simulink model "VoiceTransmissionBaseband"  (R2018a)
settings: Solver=VariableStepAuto  StartTime=0.0  StopTime=6  RelTol=1e-3
libraries: dspmathops x3, commanabbnd3 x2, dspvision x2, phasedtxrxlib x2, commchan3 x1, dspsnks4 x1, commrflib2 x1
settings Model: Creator=ASUS  LastModifiedBy=ASUS

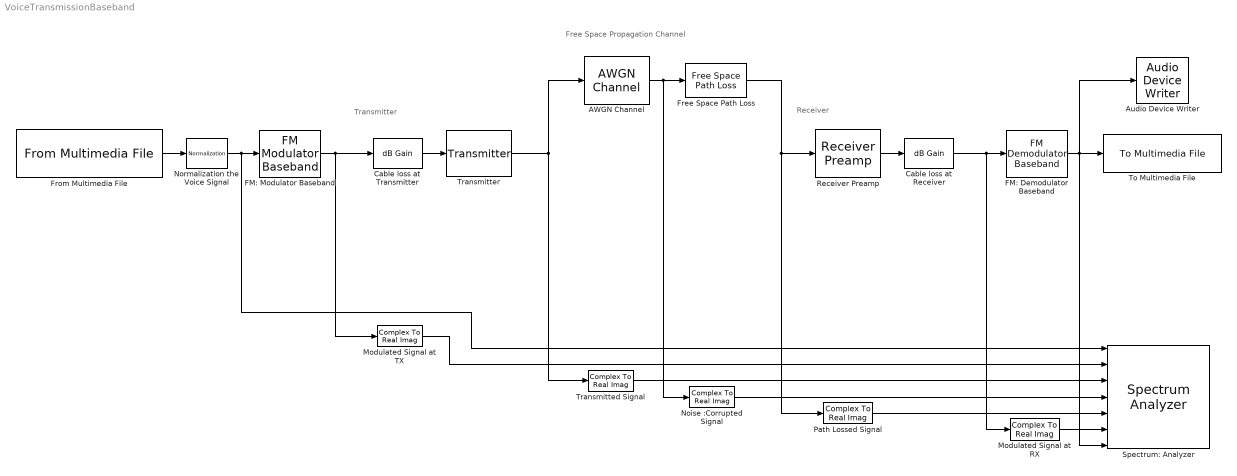
== system VoiceTransmissionBaseband ==
  note: Free Space Propagation Channel
  note: Receiver
  note: Transmitter
  AWGN Channel : commchan3/AWGN Channel  InputProcessing=Columns as channels (frame based)  seed=67  noiseMode="Signal to noise ratio  (Eb/No)"  EbNodB=-5  EsNodB=10  SNRdB=10  bitsPerSym=1  Ps=1  Tsym=1  variance=1
  Audio Device Writer : dspsnks4/Audio Device Writer  Driver=DirectSound  Device=Default  InheritSampleRate=on  SampleRate=44100  BitDepth=16-bit integer  BufferSize=4096  NumBuffers=10  DefaultOutputChannelMapping=on  OutputChannelMapping=1:2  OutputNumUnderrunSamples=off  DriverIdx=1  DeviceWarnFlag=''
  Cable loss at Receiver : dspmathops/dB Gain  dB=-4  intype=Amplitude
      settings: SourceProductName=DSP System Toolbox  SourceProductBaseCode=DS
  Cable loss at Transmitter : dspmathops/dB Gain  dB=-3  intype=Amplitude
      settings: SourceProductName=DSP System Toolbox  SourceProductBaseCode=DS
  "FM: Demodulator Baseband " : commanabbnd3/FM Demodulator Baseband   FrequencyDeviation=3999  SimulateUsing=Interpreted execution
      settings: SourceProductName=Communications System Toolbox  SourceProductBaseCode=CM
  FM: Modulator Baseband : commanabbnd3/FM Modulator Baseband  FrequencyDeviation=3999  SimulateUsing=Interpreted execution
      settings: SourceProductName=Communications System Toolbox  SourceProductBaseCode=CM
  Free Space Path Loss : commrflib2/Free Space Path Loss  mode=Decibels  dB=214.624  d=0.100  fc=1920
      settings: SourceProductName=Communications System Toolbox  SourceProductBaseCode=CM
  From Multimedia File : dspvision/From Multimedia File  inputFilename=C:\Users\ASUS\Desktop\GitRepos\RF-Propagation-Model\RFPL Modelling\code\voice.wav  loop=on  numPlays=inf  outputStreams=Audio only  videoDataType=single  audioDataType=double  inheritSampleTime=on  userDefinedSampleTime=1/30  noAudioOutput=off  isIntensityVideo=off  fourcc=RGB  colorVideoFormat=Separate color signals  outputEOF=off  dataOrg=Column-major  audioFrameSize=1024  computeAudioFrameSize=off  outSamplingMode=Sample based
      settings: SourceProductBaseCode=VP
  Modulated Signal at TX : ComplexToRealImag  Output=Real
  Modulated Signal at RX : ComplexToRealImag  Output=Real
  Noise :Corrupted Signal : ComplexToRealImag  Output=Real
  Normalization the Voice Signal : dspmathops/Normalization  NormType=2-norm  Bias=1e-10  NormOver=Each column  Dimension=1  roundingMode=Floor  overflowMode=off  accumDataTypeStr=Inherit: Same as product output  accumLastDataTypeStr=Inherit: Same as product output  outputDataTypeStr=Inherit: Same as product output  outputMin=[]  outputMax=[]  outputLastDataTypeStr=Inherit: Same as product output
      settings: SourceProductName=DSP System Toolbox
  Path Lossed Signal : ComplexToRealImag  Output=Real
  Receiver Preamp : phasedtxrxlib/Receiver Preamp  Gain=24.77  LossFactor=0  NoiseMethod=Noise temperature  NoiseFigure=0  ReferenceTemperature=290  SampleRateFromInputCheckbox=on  SampleRate=1e6  NoisePower=0  EnableInputPort=off  PhaseNoiseInputPort=off  SeedSource=Property  Seed=randi(65535,1)  SimulateUsing=Interpreted execution
      settings: SourceProductName=Phased Array System Toolbox  SourceProductBaseCode=AR
  Spectrum: Analyzer : SpectrumAnalyzer  NumInputPorts=7
  To Multimedia File : dspvision/To Multimedia File  outputFilename=C:\Users\ASUS\Desktop\GitRepos\RF-Propagation-Model\RFPL Modelling\code\output.wav  streamSelection=Audio only  videoCompressor=None (uncompressed)  audioCompressor=None (uncompressed)  imagePorts=Separate color signals  fileType=WAV  audioDatatype=16-bit integer  fourcc=RGB  videoQuality=75  mj2000CompFactor=10
      settings: SourceProductName=Computer Vision System Toolbox  SourceProductBaseCode=VP
  "Transmitted Signal " : ComplexToRealImag  Output=Real
  Transmitter : phasedtxrxlib/Transmitter  PeakPower=50000  Gain=30  LossFactor=0  InUseOutputPort=off  CoherentOnTransmit=on  PhaseNoiseOutputPort=off  SeedSource=Property  Seed=randi(65535,1)  SimulateUsing=Interpreted execution
      settings: SourceProductName=Phased Array System Toolbox  SourceProductBaseCode=AR
  wires:
  FM: Modulator Baseband/1 -> Modulated Signal at TX/1, Cable loss at Transmitter/1
  Cable loss at Receiver/1 -> "FM: Demodulator Baseband "/1, Modulated Signal at RX/1
  Cable loss at Transmitter/1 -> Transmitter/1
  Receiver Preamp/1 -> Cable loss at Receiver/1
  Noise :Corrupted Signal/1 -> Spectrum: Analyzer/4
  Modulated Signal at TX/1 -> Spectrum: Analyzer/2
  "Transmitted Signal "/1 -> Spectrum: Analyzer/3
  Path Lossed Signal/1 -> Spectrum: Analyzer/5
  AWGN Channel/1 -> Free Space Path Loss/1, Noise :Corrupted Signal/1
  "FM: Demodulator Baseband "/1 -> Spectrum: Analyzer/7, To Multimedia File/1, Audio Device Writer/1
  Transmitter/1 -> "Transmitted Signal "/1, AWGN Channel/1
  From Multimedia File/1 -> Normalization the Voice Signal/1
  Free Space Path Loss/1 -> Path Lossed Signal/1, Receiver Preamp/1
  Normalization the Voice Signal/1 -> Spectrum: Analyzer/1, FM: Modulator Baseband/1
  Modulated Signal at RX/1 -> Spectrum: Analyzer/6
